simulink model "asbCubeSat"  (R2020a)
settings: Solver=ode3  StartTime=0.0  StopTime=86400*365.25*1  FixedStep=CubeSatTimeStep  RelTol=1e-3  EnableMultiTasking=on
PreLoadFcn:
  | if ~builtin('license','test','Virtual_Reality_Toolbox')
  |     assignin('base','variantVisualization',0)
  | end
PostLoadFcn:
  | ATM_Model=3 %
InitFcn:
  | if evalin('base', 'exist(''variantVisualization'',''var'')') && ...
  |         evalin('base', 'variantVisualization == 1')
  |     if ~builtin('license','checkout','Virtual_Reality_Toolbox')
  |         error(message('aeroblks_cubesat:cubesat:licenseFailAnim'));
  |     end
  | end
  | 
  | if ~evalin('base','exist(''CubeSatTimeStep'')')
  |     assignin('base','CubeSatTimeStep',1);
  | end
StopFcn:
  | %save('./work/simulation/alt_km_simulation.mat','alt_km_simulation','-v7.3')
  | 
  | save( ['./work/simulation/alt_km_simulation','_a_',get_param('asbCubeSat/Edit Initial Orbit and Attitude', 'a'), '_Area_', sprintf('%.4f',vehicle.Area),'.mat'],'alt_km_simulation','-v7.3')
undefined symbols (not defined in the file): CubeSatTimeStep, initCond, magnitude, Solar_Activity, vehicle
libraries: aerolibutil x12, aerolibatmos2 x6, aerolibconvert2 x3, simulink x2, asbCubeSatEnvironmentLib x1, SignalEditorBlockLib x1, sharedutil x1, asbCubeSatActuatorsLib x1, asbCubeSatSensorsLib x1, asbCubeSatDynamicsLib x1, asbCubeSatFSWLib x1, aerolibobsolete x1
(part 2 of 2)

== system asbCubeSat/Visualization/Virtual Reality World/Compute Earth Rotation Rate/Quaternion to VRML ==
  q : Inport
  Demux : Demux
  Gain : Gain  Gain=2
  Gain3 : Gain  Gain=[-1 1 1 1]
  Mux : Mux
  Selector : Selector  InputPortWidth=4  IndexOptions=Index vector (dialog)  Indices=[2 4 3 1]  OutputSizes=1
  Trigonometric Function : Trigonometry  Operator=acos
  AxisAngle : Outport  VectorParamsAs1DForOutWhenUnconnected=off
  wires:
  Demux/4 -> Mux/4
  Demux/3 -> Mux/3
  Demux/2 -> Mux/2
  Gain/1 -> Mux/1
  Selector/1 -> Gain3/1
  Gain3/1 -> AxisAngle/1
  q/1 -> Demux/1
  Mux/1 -> Selector/1
  Trigonometric Function/1 -> Gain/1
  Demux/1 -> Trigonometric Function/1

== system asbCubeSat/Visualization/Virtual Reality World/Compute Umbra Translation/unitVec ==
  I : Inport
  Divide : Product  Inputs=*/
  Dot Product : DotProduct  InputSameDT=on  OutDataTypeStr=Inherit: Inherit via internal rule
  Sqrt : Sqrt  SaturateOnIntegerOverflow=on
  O : Outport  VectorParamsAs1DForOutWhenUnconnected=off
  wires:
  Dot Product/1 -> Sqrt/1
  I/1 -> Divide/1, Dot Product/1, Dot Product/2
  Divide/1 -> O/1
  Sqrt/1 -> Divide/2

== system asbCubeSat/Visualization/Virtual Reality World/Sat Position to VRML/ECEF to VRML ==
  M : Inport  PortDimensions=3
  Selector : Selector  InputPortWidth=3  IndexOptions=Index vector (dialog)  Indices=[2 3 1]  OutputSizes=1
  VR : Outport  PortDimensions=3  VectorParamsAs1DForOutWhenUnconnected=off
  wires:
  M/1 -> Selector/1
  Selector/1 -> VR/1

== system asbCubeSat/Visualization/Virtual Reality World/Sun Position to VRML/ECEF to VRML ==
  M : Inport  PortDimensions=3
  Selector : Selector  InputPortWidth=3  IndexOptions=Index vector (dialog)  Indices=[2 3 1]  OutputSizes=1
  VR : Outport  PortDimensions=3  VectorParamsAs1DForOutWhenUnconnected=off
  wires:
  M/1 -> Selector/1
  Selector/1 -> VR/1

== system asbCubeSat/External Forces and Torques/Perturbations Due to Atmospheric Drag/Subsystem3/NRLMSISE-00 Atmosphere Model/Subsystem ==
  In1 : Inport
  Anomalous oxygen number density : Terminator
  Demux : Demux  Outputs=9
  Density of Ar : Terminator
  Density of H : Terminator
  Density of He : Terminator
  Density of N : Terminator
  Density of N2 : Terminator
  Density of O : Terminator
  Density of O2 : Terminator
  Reshape : Reshape
  Total mass density : Outport
  wires:
  Demux/5 -> Density of Ar/1
  Demux/2 -> Density of O/1
  Demux/1 -> Density of He/1
  Demux/7 -> Density of H/1
  Demux/8 -> Density of N/1
  Demux/3 -> Density of N2/1
  Demux/9 -> Anomalous oxygen number density/1
  Demux/4 -> Density of O2/1
  In1/1 -> Demux/1
  Demux/6 -> Reshape/1  "Total mass density"
  Reshape/1 -> Total mass density/1  "Total mass density"

== system asbCubeSat/External Forces and Torques/Perturbations Due to Atmospheric Drag/Subsystem3/NRLMSISE-00 Atmosphere Model Solar/Subsystem ==
  year : Inport
  DOY : Inport  Port=2
  1-D Lookup Table : Lookup_n-D  NumberOfTableDimensions=1  BreakpointsForDimension1=Solar_Activity(:,1)  Table=Solar_Activity(:,2)  InternalRulePriority=Speed  RndMeth=Simplest  InputSameDT=on
  Ap Lookup Table : Lookup_n-D  NumberOfTableDimensions=1  BreakpointsForDimension1=Solar_Activity(:,1)  Table=Solar_Activity(:,3)  InternalRulePriority=Speed  RndMeth=Simplest  InputSameDT=on
  MATLAB Function : MATLAB Function  TreatAsAtomicUnit=on
  MATLAB Function2 : MATLAB Function  TreatAsAtomicUnit=on
  Out1 : Outport
  Ap_vec : Outport  Port=2
  wires:
  DOY/1 -> MATLAB Function/2(DOY)
  Ap Lookup Table/1 -> MATLAB Function2/1(Ap)
  MATLAB Function/1(Year_deci) -> Ap Lookup Table/1, 1-D Lookup Table/1
  MATLAB Function2/1(Ap_vec) -> Ap_vec/1
  year/1 -> MATLAB Function/1(year)
  1-D Lookup Table/1 -> Out1/1

== system asbCubeSat/External Forces and Torques/Perturbations Due to Atmospheric Drag/Subsystem3/NRLMSISE-00 Atmosphere Model Solar/Subsystem1 ==
  In1 : Inport
  Anomalous oxygen number density : Terminator
  Demux : Demux  Outputs=9
  Density of Ar : Terminator
  Density of H : Terminator
  Density of He : Terminator
  Density of N : Terminator
  Density of N2 : Terminator
  Density of O : Terminator
  Density of O2 : Terminator
  Reshape3 : Reshape
  Total mass density : Outport
  wires:
  Demux/5 -> Density of Ar/1
  Demux/2 -> Density of O/1
  Demux/1 -> Density of He/1
  Demux/7 -> Density of H/1
  Demux/8 -> Density of N/1
  Demux/3 -> Density of N2/1
  Demux/9 -> Anomalous oxygen number density/1
  Demux/4 -> Density of O2/1
  In1/1 -> Demux/1
  Demux/6 -> Reshape3/1  "Total mass density"
  Reshape3/1 -> Total mass density/1  "Total mass density"

== matlab function asbCubeSat/External Forces and Torques/Perturbations Due to Atmospheric Drag/MATLAB Function1 ==
  data: Julian_day input; year output; doy output; sec output
function [year, doy, sec] = Julian2YDSv2(Julian_day) 

% convert to calender date,time (UTC)
t = datetime(Julian_day,'convertfrom','juliandate');
t_vec = datevec(t);

% output year, sec
year = t_vec(1);
sec = t_vec(4)*3600 + t_vec(5)*60 + t_vec(6);


% define DOY of the 1st day in a month (normal year)
d = zeros(1,12);
d(1) = 1; d(2) = 32;
d(3) = 60; d(4) = 91;
d(5) = 121; d(6) = 152;
d(7) = 182; d(8) = 213;
d(9) = 244; d(10) = 274;
d(11) = 305; d(12) = 335;

% define DOY of the 1st day in a month (leap year)
dL = zeros(1,12);
dL(1) = 1; dL(2) = 32;
dL(3) = 61; dL(4) = 92;
dL(5) = 122; dL(6) = 153;
dL(7) = 183; dL(8) = 214;
dL(9) = 245; dL(10) = 275;
dL(11) = 306; dL(12) = 336;

doy = 0;
% output Day of Year
    % normal year
    if mod(t_vec(1),4) ~= 0;     
        doy = d(t_vec(2)) + t_vec(3) - 1;
    end
    
    % leap year
    if mod(t_vec(1),4) == 0; 
        doy = dL(t_vec(2)) + t_vec(3) - 1;
    end

end

== matlab function asbCubeSat/External Forces and Torques/Perturbations Due to Atmospheric Drag/NRLMSISE-00 Atmosphere Model Solar/MATLAB Function ==
  data: year input; Year_deci output; DOY input
function Year_deci = YD2Ydecimal(year, DOY)

day = 0;
% normal year
    if mod(year,4) ~= 0;     
        day = 365;
    else
        day = 366;
    end
    
Year_deci = year + DOY/day;

end

== stateflow chart asbCubeSat/External Forces and Torques/Thruster/Chart ==
  state InActive
    thruster_x=0;
    thruster_y=0;
    thruster_z=0;
  state ReActive
    thruster_x=inThrustForce_x;
    thruster_y=inThrustForce_y;
    thruster_z=inThrustForce_z;
  (default) -> InActive
  InActive -> ReActive : [inOneCycle==true && inActivateThruster]
  ReActive -> InActive : [after(parDurationMin*60,sec)]
  data: thruster_x output; thruster_y output; thruster_z output; inOneCycle input; inThrustForce_x input; inThrustForce_y input; inThrustForce_z input; inActivateThruster input; parDurationMin input

== matlab function asbCubeSat/External Forces and Torques/Perturbations Due to Atmospheric Drag/NRLMSISE-00 Atmosphere Model Solar/MATLAB Function2 ==
  data: Ap input; Ap_vec output
function Ap_vec = Multi_Ap(Ap)

Ap_vec = repmat(Ap,1,7);

== matlab function asbCubeSat/External Forces and Torques/Perturbations Due to Atmospheric Drag/Subsystem3/NRLMSISE-00 Atmosphere Model Solar/Subsystem/MATLAB Function ==
  data: year input; Year_deci output; DOY input
function Year_deci = YD2Ydecimal(year, DOY)

day = 0;
% normal year
    if mod(year,4) ~= 0;     
        day = 365;
    else
        day = 366;
    end
    
Year_deci = year + DOY/day;

end

== matlab function asbCubeSat/External Forces and Torques/Perturbations Due to Atmospheric Drag/Subsystem3/NRLMSISE-00 Atmosphere Model Solar/Subsystem/MATLAB Function2 ==
  data: Ap input; Ap_vec output
function Ap_vec = Multi_Ap(Ap)

Ap_vec = repmat(Ap,1,7);
